simulink model "ControlDistributor"  (R2022a)
settings: Solver=VariableStepAuto  StartTime=0.0  StopTime=10.0  RelTol=1e-3
model workspace (MAT data in the model file):
  CM = 1.779e-07
  CR = 1148
  CT = 1.105e-05
  J = [0.0211  0  0; 0  0.0219  0; 0  0  0.0366]
  JPR = 0.0001287
  Tm = 0.05
  d = 0.225
  m = 1.4
  sqrt22 = 0.70710678
  wb = -141.4
settings Model: Creator=Lenovo  LastModifiedBy=Lenovo

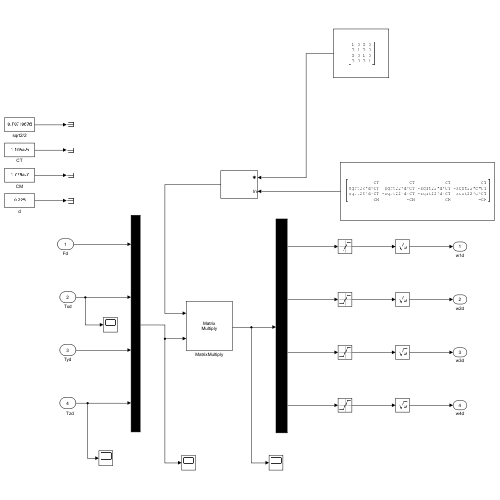
[thumbnail: Simulink's stored preview of the top-level diagram]
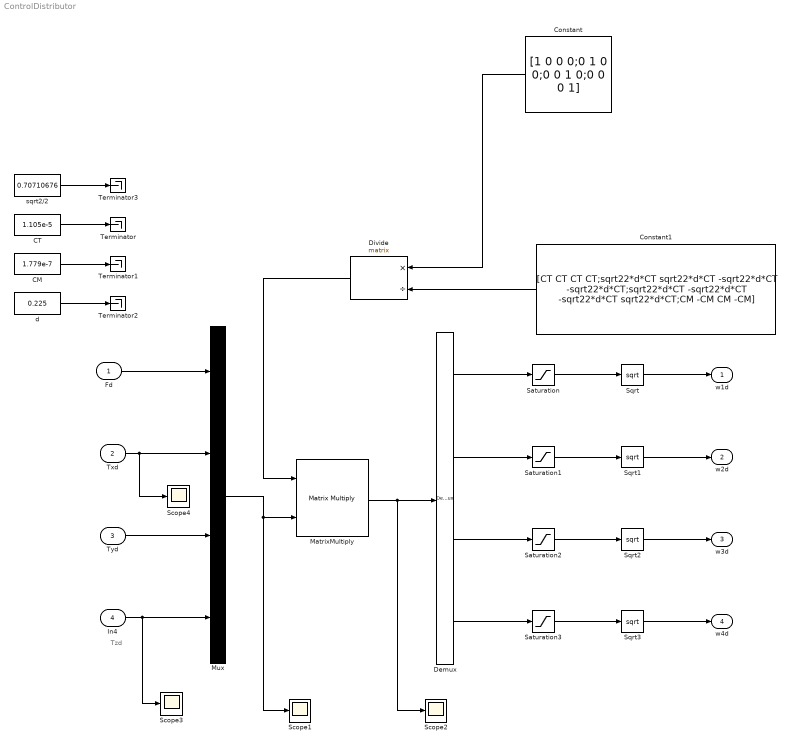
== system ControlDistributor ==
  note: Tzd
  Fd : Inport
  Txd : Inport  Port=2
  Tyd : Inport  Port=3
  In4 : Inport  Port=4
  CM : Constant  Value=1.779e-7
  CT : Constant  Value=1.105e-5
  Constant : Constant  Value=[1 0 0 0;0 1 0 0;0 0 1 0;0 0 0 1]
  Constant1 : Constant  Value=[CT CT CT CT;sqrt22*d*CT sqrt22*d*CT -sqrt22*d*CT -sqrt22*d*CT;sqrt22*d*CT -sqrt22*d*CT -sqrt22*d*CT sqrt22*d*CT;CM -CM CM -CM]
  Demux : Demux
  Divide : Product  Inputs=*/  Multiplication=Matrix(*)
  MatrixMultiply : Product  Multiplication=Matrix(*)
  Mux : Mux
  Saturation{,1..3} (4 alike) : Saturate
  Scope{1..4} (4 alike) : Scope
  Sqrt{,1..3} (4 alike) : Sqrt
  Terminator{,1..3} (4 alike) : Terminator
  d : Constant  Value=0.225
  sqrt2/2 : Constant  Value=0.70710676
  w1d : Outport
  w2d : Outport  Port=2
  w3d : Outport  Port=3
  w4d : Outport  Port=4
  wires:
  Fd/1 -> Mux/1
  Tyd/1 -> Mux/3
  Txd/1 -> Scope4/1, Mux/2
  In4/1 -> Scope3/1, Mux/4
  MatrixMultiply/1 -> Scope2/1, Demux/1
  Mux/1 -> Scope1/1, MatrixMultiply/2
  Constant/1 -> Divide/1
  CT/1 -> Terminator/1
  CM/1 -> Terminator1/1
  d/1 -> Terminator2/1
  sqrt2/2/1 -> Terminator3/1
  Demux/1 -> Saturation/1
  Saturation/1 -> Sqrt/1
  Sqrt/1 -> w1d/1
  Sqrt1/1 -> w2d/1
  Saturation1/1 -> Sqrt1/1
  Demux/2 -> Saturation1/1
  Saturation2/1 -> Sqrt2/1
  Sqrt2/1 -> w3d/1
  Sqrt3/1 -> w4d/1
  Saturation3/1 -> Sqrt3/1
  Demux/4 -> Saturation3/1
  Demux/3 -> Saturation2/1
  Constant1/1 -> Divide/2
  Divide/1 -> MatrixMultiply/1
